simulink model "fbl_ctrl"  (R2021a)
settings: Solver=VariableStepAuto  StartTime=0.0  StopTime=tf  FixedStep=simstep  RelTol=1e-3
values from neighbouring files (symbols this model uses):
  apply_noise = 1    [fbl.m]
  e = 0.01    [main.m]
  f = 0.0045    [main.m]
  k_fbl = 4.35    [fbl.m]
  noise_a = -20e-7    (= -2e-06)    [main.m]
  noise_b = -50e-7    (= -5e-06)    [main.m]
  r = 0    [main.m]
  Ts = 0.02    [main.m]
  x0 = [950; 550; 6e-4]    [main.m]
  x10 = 1000    [main.m]
  x20 = 550    [main.m]
libraries: simulink x1
settings Model: Creator=micma  LastModifiedBy=micma

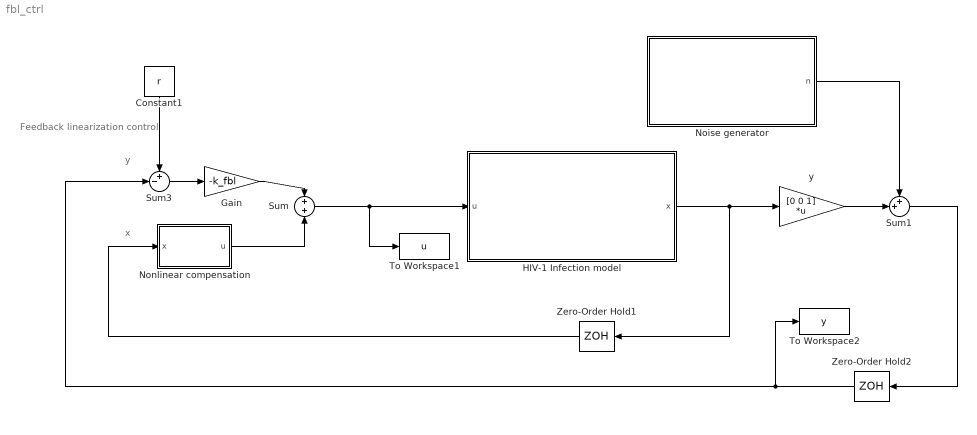
== system fbl_ctrl ==
  note: y
  note: Feedback linearization
      | control
  note: x
  Constant1 : Constant  Value=r
  Gain : Gain  Gain=-k_fbl
  HIV-1 Infection model : Subsystem
  Noise generator : Subsystem
  Nonlinear compensation : Subsystem
  Sum : Sum
  Sum1 : Sum  Inputs=++|
  Sum3 : Sum  Inputs=+-|
  To Workspace1 : ToWorkspace  VariableName=u  SaveFormat=Timeseries  SampleTime=-1
  To Workspace2 : ToWorkspace  VariableName=y  SaveFormat=Timeseries  SampleTime=-1
  Zero-Order Hold1 : ZeroOrderHold  SampleTime=Ts
  Zero-Order Hold2 : ZeroOrderHold  SampleTime=Ts
  y : Gain  Gain=[0 0 1]  Multiplication=Matrix(K*u)
  wires:
  Zero-Order Hold1/1 -> Nonlinear compensation/1(x)
  Sum3/1 -> Gain/1
  Nonlinear compensation/1(u) -> Sum/2
  Gain/1 -> Sum/1
  HIV-1 Infection model/1(x) -> y/1, Zero-Order Hold1/1
  Sum/1 -> HIV-1 Infection model/1(u), To Workspace1/1
  Constant1/1 -> Sum3/1
  Noise generator/1(n) -> Sum1/1
  y/1 -> Sum1/2
  Sum1/1 -> Zero-Order Hold2/1
  Zero-Order Hold2/1 -> To Workspace2/1, Sum3/2

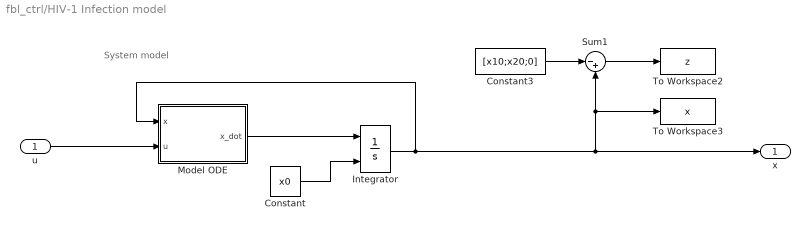
== system fbl_ctrl/HIV-1 Infection model ==
  note: System model
  u : Inport
  Constant : Constant  Value=x0
  Constant3 : Constant  Value=[x10;x20;0]
  Integrator : Integrator  InitialConditionSource=external
  Model ODE : MATLAB Function  TreatAsAtomicUnit=on
  Sum1 : Sum  Inputs=|-+
  To Workspace2 : ToWorkspace  VariableName=z  SaveFormat=Timeseries  SampleTime=-1
  To Workspace3 : ToWorkspace  VariableName=x  SaveFormat=Timeseries  SampleTime=-1
  x : Outport
  wires:
  Model ODE/1(x_dot) -> Integrator/1
  Constant/1 -> Integrator/2
  u/1 -> Model ODE/2(u)
  Constant3/1 -> Sum1/1
  Sum1/1 -> To Workspace2/1
  Integrator/1 -> x/1, To Workspace3/1, Sum1/2, Model ODE/1(x)

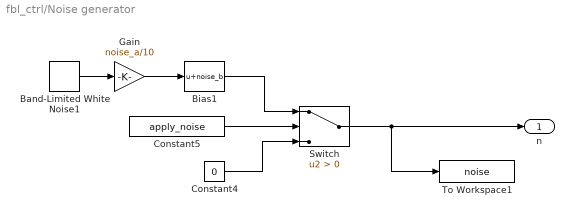
== system fbl_ctrl/Noise generator ==
  Band-Limited White Noise1 : simulink/Sources/Band-Limited White Noise  Cov=[.1]  Ts=Ts*0.1  seed=[23341]
  Bias1 : Bias  Bias=noise_b
  Constant4 : Constant  Value=0
  Constant5 : Constant  Value=apply_noise
  Gain : Gain  Gain=noise_a/10
  Switch : Switch  Criteria=u2 > Threshold
  To Workspace1 : ToWorkspace  VariableName=noise  SaveFormat=Timeseries  SampleTime=-1
  n : Outport
  wires:
  Constant5/1 -> Switch/2
  Constant4/1 -> Switch/3
  Switch/1 -> n/1, To Workspace1/1
  Bias1/1 -> Switch/1
  Band-Limited White Noise1/1 -> Gain/1
  Gain/1 -> Bias1/1

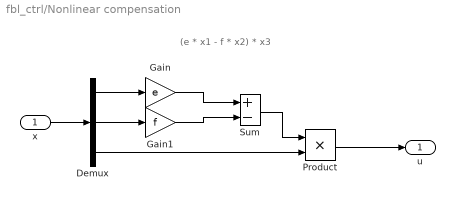
== system fbl_ctrl/Nonlinear compensation ==
  note: (e * x1 - f * x2) * x3
  x : Inport
  Demux : Demux  Outputs=3
  Gain : Gain  Gain=e
  Gain1 : Gain  Gain=f
  Product : Product
  Sum : Sum  Inputs=+-
  u : Outport
  wires:
  x/1 -> Demux/1
  Demux/1 -> Gain/1
  Demux/2 -> Gain1/1
  Gain/1 -> Sum/1
  Gain1/1 -> Sum/2
  Sum/1 -> Product/1
  Demux/3 -> Product/2
  Product/1 -> u/1

== matlab function fbl_ctrl/HIV-1 Infection model/Model ODE ==
  data: x input; u input; x_dot output; params parameter
function x_dot = ode(x, u, params)
x_dot = modelODE(x, u, params);
end
